simulink model "Model_40_01_1"  (R2024b)
settings: Solver=VariableStepAuto  StartTime=0.0  StopTime=50  FixedStep=0.02  RelTol=tol_rel  AbsTol=tol_abs
undefined symbols (not defined in the file): z03
settings Model: Creator=eddyp  LastModifiedBy=ricki
settings DataIOCC: OutputOption=SpecifiedOutputTimes  OutputTimes=t2_d

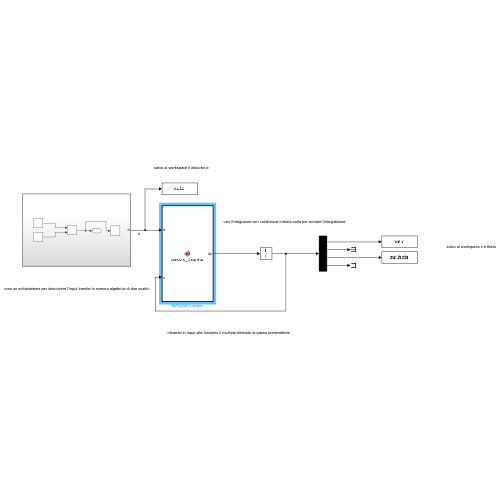
[thumbnail: Simulink's stored preview of the top-level diagram]
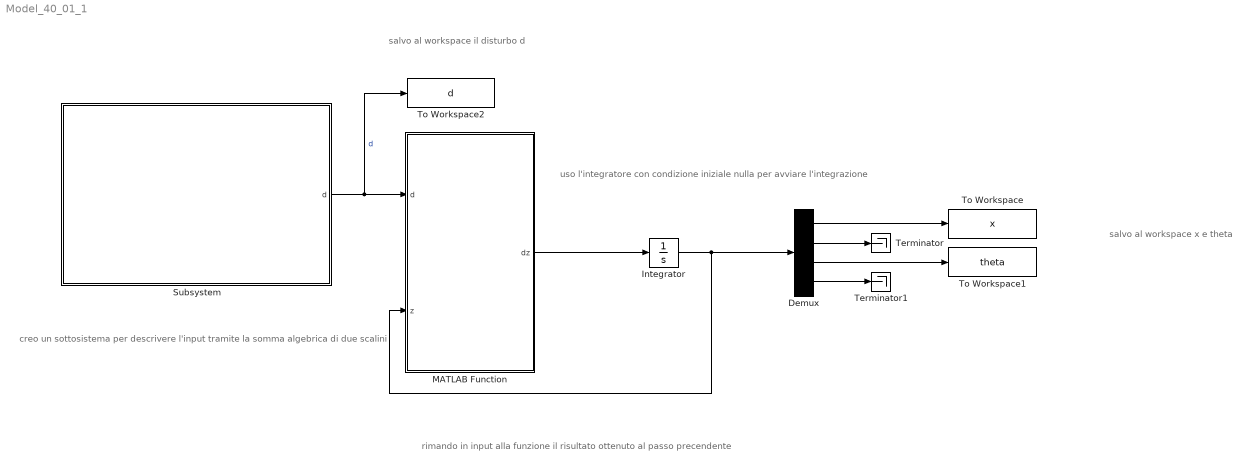
== system Model_40_01_1 ==
  note: rimando in input alla funzione il risultato ottenuto al passo precendente
  note: creo un sottosistema per descrivere l'input tramite la somma algebrica di due scalini
  note: uso l'integratore con condizione iniziale nulla per avviare l'integrazione
  note: salvo al workspace il disturbo d
  note: salvo al workspace x e theta
  Demux : Demux
  Integrator : Integrator  InitialCondition=z03  AbsoluteTolerance=1e-4
  MATLAB Function : MATLAB Function  TreatAsAtomicUnit=on
  Subsystem : Subsystem
  Terminator : Terminator
  Terminator1 : Terminator
  To Workspace : ToWorkspace  VariableName=x
      settings: Save2DSignal=2-D array (concatenate along first dimension)
  To Workspace1 : ToWorkspace  VariableName=theta
      settings: Save2DSignal=2-D array (concatenate along first dimension)
  To Workspace2 : ToWorkspace  VariableName=d
      settings: Save2DSignal=2-D array (concatenate along first dimension)
  wires:
  Subsystem/1(d) -> To Workspace2/1, MATLAB Function/1(d)  "d"
  MATLAB Function/1(dz) -> Integrator/1
  Integrator/1 -> Demux/1, MATLAB Function/2(z)
  Demux/2 -> Terminator/1
  Demux/4 -> Terminator1/1
  Demux/1 -> To Workspace/1
  Demux/3 -> To Workspace1/1

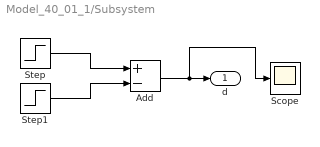
== system Model_40_01_1/Subsystem ==
  Add : Sum  Inputs=+-
  Scope : Scope
  Step : Step  SampleTime=0
  Step1 : Step  Time=3  SampleTime=0
  d : Outport
  wires:
  Step/1 -> Add/1
  Step1/1 -> Add/2
  Add/1 -> Scope/1, d/1

== matlab function Model_40_01_1/MATLAB Function ==
  data: d input; dz output; z input; lab1P parameter
function dz = pendolo_dinamica(d, z, lab1P)
% la funzione riceve in input il disturbo d e lo stato z e restituisce lo
% stato derivato

ii=0; % controllo posto a zero , corrente nulla

den=(lab1P.I0*lab1P.I2 - lab1P.I1^2*cos(z(3))^2 + lab1P.I2*lab1P.M);
dz=[z(2); % derivando z alla riga due ottengo x_dot_dot 
    -(- lab1P.g*sin(z(3))*lab1P.I1^2*cos(z(3)) + lab1P.I2*sin(z(3))*lab1P.I1*z(4)^2 + lab1P.b*lab1P.I1*z(4)*cos(z(3)) - lab1P.alpha1*d*lab1P.I1*cos(z(3))^2 + lab1P.I2*lab1P.alpha0*d - lab1P.I2*lab1P.alpham*ii + lab1P.I2*lab1P.c*z(2))/den;
    z(4); % derivando z alla riga quattro ottengo theta_dot_dot 
    -(lab1P.I0*lab1P.b*z(4) + lab1P.M*lab1P.b*z(4) - lab1P.I0*lab1P.I1*lab1P.g*sin(z(3)) - lab1P.I1*lab1P.M*lab1P.g*sin(z(3)) - lab1P.I0*lab1P.alpha1*d*cos(z(3)) + lab1P.I1*lab1P.alpha0*d*cos(z(3)) - lab1P.M*lab1P.alpha1*d*cos(z(3)) - lab1P.I1*lab1P.alpham*ii*cos(z(3)) + lab1P.I1*lab1P.c*z(2)*cos(z(3)) + lab1P.I1^2*z(4)^2*cos(z(3))*sin(z(3)))/den];

end
